simulink model "Usrednjeni_model"  (R2023b)
settings: Solver=ode23t  StartTime=0.0  StopTime=0.001  MaxStep=2.0  RelTol=1e-3
model workspace (MAT data in the model file):
  Upv = 0.5
values from neighbouring files (symbols this model uses):
  pv_data =     [CNC110X69-5.mat]
undefined symbols (not defined in the file or in its folder): Ci, Cu, Ipv0, L, R, RL, T, Uoc_max
libraries: simulink x3, spsBistableLib x1
settings Model: Creator=teo  LastModifiedBy=teo

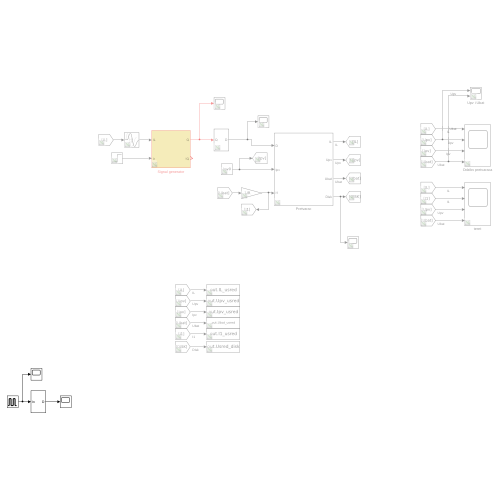
[thumbnail: Simulink's stored preview of the top-level diagram]
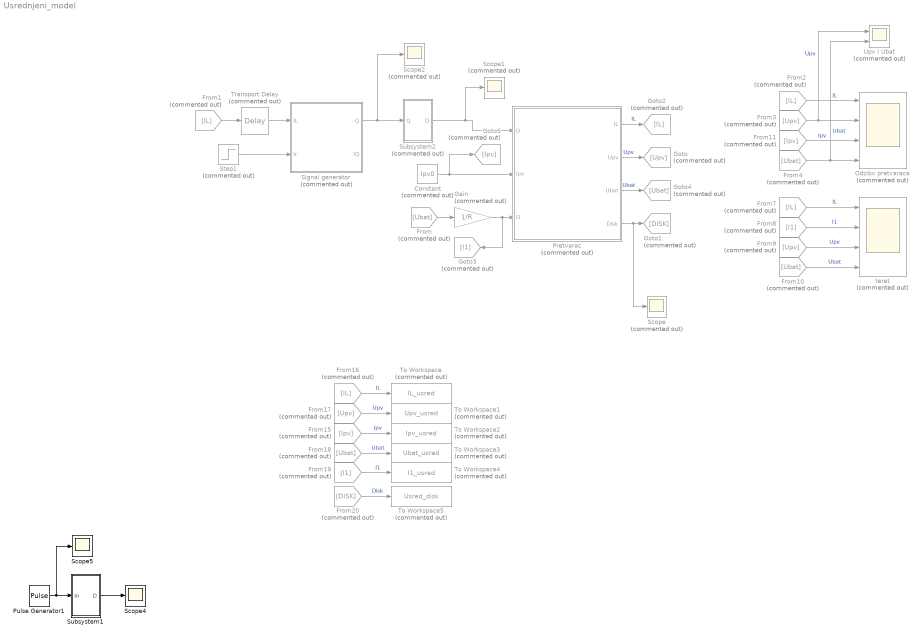
== system Usrednjeni_model ==
  Constant : Constant  Commented=on  Value=Ipv0
  From{,4,10,18} (4 alike) : From  Commented=on  GotoTag=Ubat
  From{1..2,7,16} (4 alike) : From  Commented=on  GotoTag=IL
  From11 : From  Commented=on  GotoTag=Ipv
  From15 : From  Commented=on  GotoTag=Ipv
  From17 : From  Commented=on  GotoTag=Upv
  From19 : From  Commented=on  GotoTag=I1
  From20 : From  Commented=on  GotoTag=DISK
  From3 : From  Commented=on  GotoTag=Upv
  From8 : From  Commented=on  GotoTag=I1
  From9 : From  Commented=on  GotoTag=Upv
  Gain : Gain  Commented=on  Gain=1/R
  Goto : Goto  Commented=on  GotoTag=Upv
  Goto1 : Goto  Commented=on  GotoTag=DISK
  Goto2 : Goto  Commented=on  GotoTag=IL
  Goto3 : Goto  Commented=on  GotoTag=I1
  Goto4 : Goto  Commented=on  GotoTag=Ubat
  Goto5 : Goto  Commented=on  GotoTag=Ipv
  Odzibv pretvaraca : Scope  Commented=on  NumInputPorts=4
  Pretvarac : Subsystem  Commented=on
  Pulse Generator1 : DiscretePulseGenerator  PulseType=Time based  Period=T  PulseWidth=50
  Scope : Scope  Commented=on
  Scope1 : Scope  Commented=on
  Scope2 : Scope  Commented=on
  Scope4 : Scope
  Scope5 : Scope
  Signal generator : Subsystem  Commented=on
  Step1 : Step  Commented=on  Time=0.002  Before=0.1  After=Ipv0 - 0.05  SampleTime=0
  Subsystem1 : Subsystem
  Subsystem2 : Subsystem  Commented=on
  To Workspace : ToWorkspace  Commented=on  VariableName=IL_usred  SaveFormat=Timeseries  SampleTime=-1
  To Workspace1 : ToWorkspace  Commented=on  VariableName=Upv_usred  SaveFormat=Timeseries  SampleTime=-1
  To Workspace2 : ToWorkspace  Commented=on  VariableName=Ipv_usred  SaveFormat=Timeseries  SampleTime=-1
  To Workspace3 : ToWorkspace  Commented=on  VariableName=Ubat_usred  SaveFormat=Timeseries  SampleTime=-1
  To Workspace4 : ToWorkspace  Commented=on  VariableName=I1_usred  SaveFormat=Timeseries  SampleTime=-1
  To Workspace5 : ToWorkspace  Commented=on  VariableName=Usred_disk  SaveFormat=Timeseries  SampleTime=-1
  Transport Delay : TransportDelay  Commented=on  DelayTime=0.0001
  Upv i Ubat : Scope  Commented=on  NumInputPorts=2
  teret : Scope  Commented=on  NumInputPorts=4
  wires:
  Pretvarac/1(IL) -> Goto2/1  "IL"
  Pretvarac/2(Upv) -> Goto/1  "Upv"
  Pretvarac/3(Ubat) -> Goto4/1  "Ubat"
  Pretvarac/4(Disk) -> Scope/1, Goto1/1
  Gain/1 -> Goto3/1, Pretvarac/3(I1)
  From/1 -> Gain/1
  From4/1 -> Upv i Ubat/2, Odzibv pretvaraca/4  "Ubat"
  From2/1 -> Odzibv pretvaraca/1  "IL"
  From3/1 -> Upv i Ubat/1, Odzibv pretvaraca/2  "Upv"
  From8/1 -> teret/2  "I1"
  From10/1 -> teret/4  "Ubat"
  From11/1 -> Odzibv pretvaraca/3  "Ipv"
  From7/1 -> teret/1  "IL"
  From9/1 -> teret/3  "Upv"
  From18/1 -> To Workspace3/1  "Ubat"
  From15/1 -> To Workspace2/1  "Ipv"
  From17/1 -> To Workspace1/1  "Upv"
  From19/1 -> To Workspace4/1  "I1"
  From16/1 -> To Workspace/1  "IL"
  From20/1 -> To Workspace5/1  "Disk"
  Step1/1 -> Signal generator/2(Ir)
  Constant/1 -> Goto5/1, Pretvarac/2(Ipv)
  Subsystem1/1(D) -> Scope4/1
  Pulse Generator1/1 -> Scope5/1, Subsystem1/1(In)
  Signal generator/1(Q) -> Scope2/1, Subsystem2/1(Q)
  Subsystem2/1(D) -> Scope1/1, Pretvarac/1(D)
  Transport Delay/1 -> Signal generator/1(IL)
  From1/1 -> Transport Delay/1

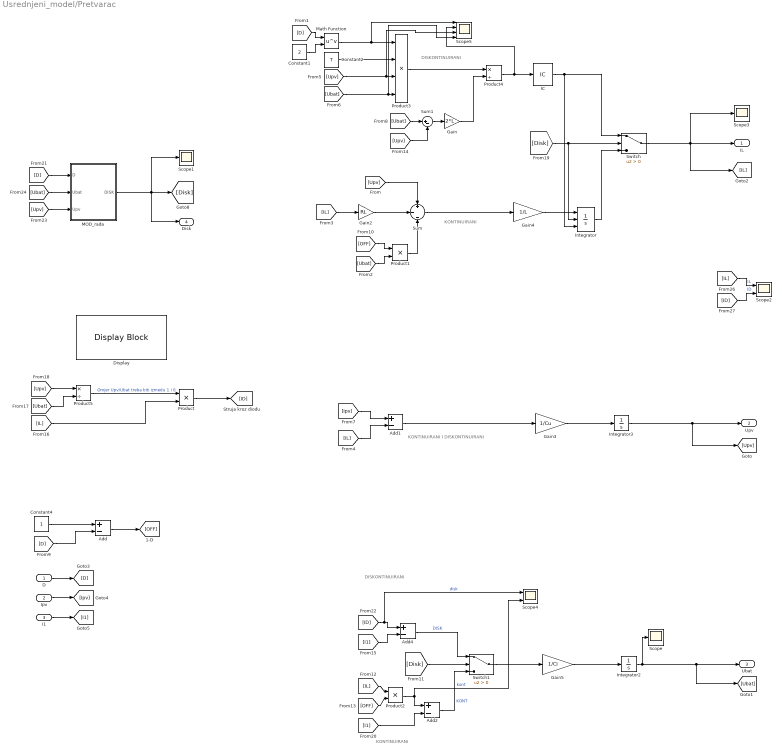
== system Usrednjeni_model/Pretvarac ==
  note: DISKONTINUIRANI
  note: KONTINUIRANI
  note: KONTINUIRANI I DISKONTINUIRANI
  note: KONTINUIRANI
  note: DISKONTINUIRANI
  D : Inport
  Ipv : Inport  Port=2
  I1 : Inport  Port=3
  Add{,1..2,4} (4 alike) : Sum  Inputs=+-
  Constant1 : Constant  Value=2
  Constant2 : Constant  Value=T
  Constant4 : Constant
  Display : DisplayBlock  LabelPosition=Bottom  Transparency=1
  Gain : Gain  Gain=2*L
  Gain2 : Gain  Gain=RL
  Gain3 : Gain  Gain=1/Cu
  Gain4 : Gain  Gain=1/L
  Gain5 : Gain  Gain=1/Ci
  IC : InitialCondition  Value=0.1
  Integrator : Integrator  ExternalReset=falling  InitialConditionSource=external  LimitOutput=on  UpperSaturationLimit=150  LowerSaturationLimit=0
  Integrator2 : Integrator  InitialCondition=0.2  UpperSaturationLimit=Uoc_max + 10  LowerSaturationLimit=0
  Integrator3 : Integrator  InitialCondition=0.1  LimitOutput=on  UpperSaturationLimit=pv_data.Voc  LowerSaturationLimit=0
  MOD_rada : Subsystem
  Math Function : Math  Operator=pow
  Product : Product
  Product1 : Product
  Product2 : Product
  Product3 : Product  Inputs=4
  Product4 : Product  Inputs=*/
  Product5 : Product  Inputs=*/
  Scope : Scope
  Scope1 : Scope
  Scope2 : Scope  NumInputPorts=2
  Scope3 : Scope
  Scope4 : Scope  NumInputPorts=2
  Scope5 : Scope  NumInputPorts=4
  Sum : Sum  Inputs=+|-|-
  Sum1 : Sum  Inputs=|+-
  Switch : Switch  Criteria=u2 > Threshold  SaturateOnIntegerOverflow=off  InputSameDT=off
  Switch1 : Switch  Criteria=u2 > Threshold  SaturateOnIntegerOverflow=off  InputSameDT=off
  IL : Outport
  Upv : Outport  Port=2
  Ubat : Outport  Port=3
  Disk : Outport  Port=4
  wires:
  I1/1 -> [I1]
  [Ipv] -> Add1/1
  D/1 -> [D]
  Ipv/1 -> [Ipv]
  [Upv] -> Sum/1
  [D] -> Add/2
  Constant4/1 -> Add/1
  Product1/1 -> Sum/3
  [OFF] -> Product1/1
  [Ubat] -> Product1/2
  [IL] -> Add1/2
  Sum/1 -> Gain4/1
  Add1/1 -> Gain3/1
  [D] -> Math Function/1
  Constant1/1 -> Math Function/2
  Math Function/1 -> Scope5/1, Product3/1
  Constant2/1 -> Product3/2
  [Upv] -> Scope5/3, Product3/3
  [Ubat] -> Scope5/4, Product3/4
  Product3/1 -> Product4/1
  [Ubat] -> Sum1/1
  [Upv] -> Sum1/2
  Sum1/1 -> Gain/1
  Gain3/1 -> Integrator3/1
  Gain/1 -> Product4/2
  Switch/1 -> Scope3/1, IL/1, [IL]
  Add/1 -> [OFF]
  Gain2/1 -> Sum/2
  [IL] -> Gain2/1
  Gain5/1 -> Integrator2/1
  [D] -> MOD_rada/1(D)
  [Upv] -> MOD_rada/3(Upv)
  [Ubat] -> MOD_rada/2(Ubat)
  Integrator3/1 -> [Upv], Upv/1
  Gain4/1 -> Integrator/1
  Integrator/1 -> Switch/3
  [Disk] -> Integrator/2, Switch/2
  [Upv] -> Product5/1
  [Ubat] -> Product5/2
  [IL] -> Product/2
  Product/1 -> [ID]
  Product5/1 -> Product/1  "Omjer Upv/Ubat treba biti izmedu 1 i 0"
  [ID] -> Scope4/1, Add4/1  "disk"
  [I1] -> Add4/2
  [IL] -> Scope2/1  "IL"
  [ID] -> Scope2/2  "ID"
  IC/1 -> Integrator/3, Switch/1
  Switch1/1 -> Gain5/1
  Add4/1 -> Switch1/1  "DISK"
  [Disk] -> Switch1/2
  [IL] -> Product2/1
  [OFF] -> Product2/2
  Product2/1 -> Add2/1, Scope4/2  "kont"
  [I1] -> Add2/2
  Add2/1 -> Switch1/3  "KONT"
  MOD_rada/1(DISK) -> Disk/1, Scope1/1, [Disk]
  Integrator2/1 -> [Ubat], Ubat/1, Scope/1
  Product4/1 -> Scope5/2, IC/1

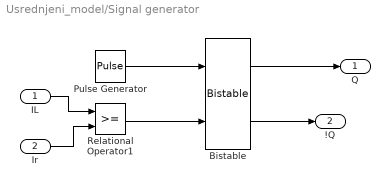
== system Usrednjeni_model/Signal generator ==
  IL : Inport
  Ir : Inport  Port=2
  Bistable : spsBistableLib/Bistable  Qpriority=Set  ic=0  Ts=0
      settings: LibrarySourceBlock=sps_lib/Control/Bistable
  Pulse Generator : DiscretePulseGenerator  PulseType=Time based  Period=T
  Relational Operator1 : RelationalOperator  OutDataTypeStr=boolean  RndMeth=Simplest  InputSameDT=off
  Q : Outport
  !Q : Outport  Port=2
  wires:
  Pulse Generator/1 -> Bistable/1
  Ir/1 -> Relational Operator1/2
  Relational Operator1/1 -> Bistable/2
  IL/1 -> Relational Operator1/1
  Bistable/2 -> !Q/1
  Bistable/1 -> Q/1

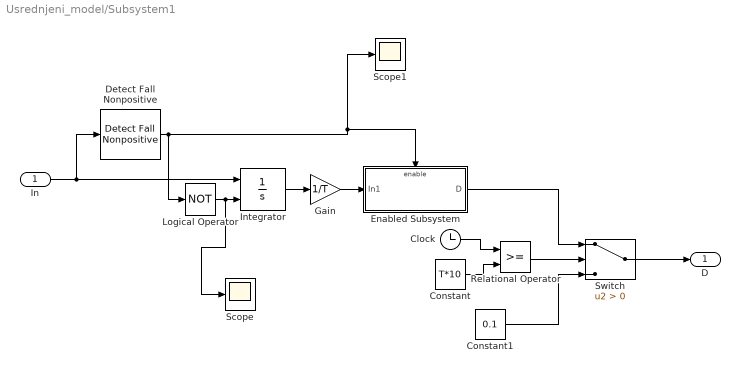
== system Usrednjeni_model/Subsystem1 ==
  In : Inport
  Clock : Clock
  Constant : Constant  Value=T*10
  Constant1 : Constant  Value=0.1
  Detect Fall Nonpositive : simulink/Logic and Bit Operations/Detect Fall Nonpositive  vinit=0  OutDataTypeStr=boolean
  Enabled Subsystem : Subsystem  TreatAsAtomicUnit=on
  Gain : Gain  Gain=1/T
  Integrator : Integrator  ExternalReset=rising
  Logical Operator : Logic  Operator=NOT  AllPortsSameDT=off  OutDataTypeStr=boolean
  Relational Operator : RelationalOperator  OutDataTypeStr=boolean  RndMeth=Simplest  InputSameDT=off
  Scope : Scope
  Scope1 : Scope
  Switch : Switch  Criteria=u2 > Threshold  SaturateOnIntegerOverflow=off  InputSameDT=off
  D : Outport
  wires:
  In/1 -> Integrator/1, Detect Fall Nonpositive/1
  Integrator/1 -> Gain/1
  Gain/1 -> Enabled Subsystem/1(In1)
  Enabled Subsystem/1(D) -> Switch/1
  Switch/1 -> D/1
  Clock/1 -> Relational Operator/1
  Constant/1 -> Relational Operator/2
  Relational Operator/1 -> Switch/2
  Constant1/1 -> Switch/3
  Detect Fall Nonpositive/1 -> Logical Operator/1, Scope1/1, Enabled Subsystem/Enable
  Logical Operator/1 -> Scope/1, Integrator/2

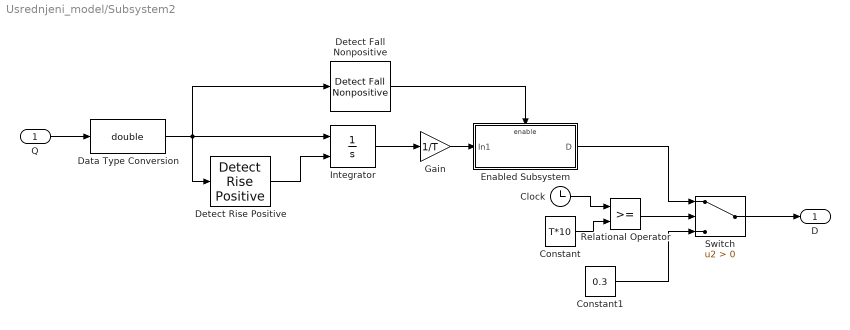
== system Usrednjeni_model/Subsystem2 ==
  Q : Inport
  Clock : Clock
  Constant : Constant  Value=T*10
  Constant1 : Constant  Value=0.3
  Data Type Conversion : DataTypeConversion  OutDataTypeStr=double  SaturateOnIntegerOverflow=off  RndMeth=Floor
  Detect Fall Nonpositive : simulink/Logic and Bit Operations/Detect Fall Nonpositive  vinit=0  OutDataTypeStr=boolean
  Detect Rise Positive : simulink/Logic and Bit Operations/Detect Rise Positive  vinit=0  OutDataTypeStr=boolean
  Enabled Subsystem : Subsystem  TreatAsAtomicUnit=on
  Gain : Gain  Gain=1/T
  Integrator : Integrator  ExternalReset=rising
  Relational Operator : RelationalOperator  OutDataTypeStr=boolean  RndMeth=Simplest  InputSameDT=off
  Switch : Switch  Criteria=u2 > Threshold  SaturateOnIntegerOverflow=off  InputSameDT=off
  D : Outport
  wires:
  Integrator/1 -> Gain/1
  Detect Rise Positive/1 -> Integrator/2
  Gain/1 -> Enabled Subsystem/1(In1)
  Detect Fall Nonpositive/1 -> Enabled Subsystem/Enable
  Enabled Subsystem/1(D) -> Switch/1
  Switch/1 -> D/1
  Clock/1 -> Relational Operator/1
  Constant/1 -> Relational Operator/2
  Relational Operator/1 -> Switch/2
  Constant1/1 -> Switch/3
  Q/1 -> Data Type Conversion/1
  Data Type Conversion/1 -> Detect Rise Positive/1, Detect Fall Nonpositive/1, Integrator/1

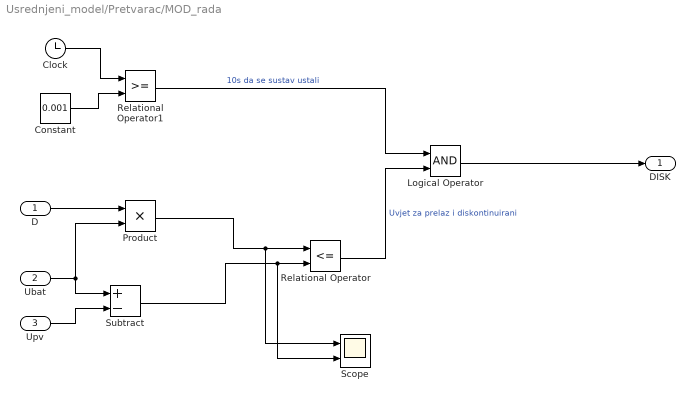
== system Usrednjeni_model/Pretvarac/MOD_rada ==
  D : Inport
  Ubat : Inport  Port=2
  Upv : Inport  Port=3
  Clock : Clock
  Constant : Constant  Value=0.001
  Logical Operator : Logic  AllPortsSameDT=off  OutDataTypeStr=boolean
  Product : Product
  Relational Operator : RelationalOperator  Operator=<=  OutDataTypeStr=boolean  RndMeth=Simplest  InputSameDT=off
  Relational Operator1 : RelationalOperator  OutDataTypeStr=boolean  RndMeth=Simplest  InputSameDT=off
  Scope : Scope  NumInputPorts=2
  Subtract : Sum  Inputs=+-
  DISK : Outport
  wires:
  Ubat/1 -> Product/2, Subtract/1
  Upv/1 -> Subtract/2
  Relational Operator1/1 -> Logical Operator/1  "10s da se sustav ustali"
  Relational Operator/1 -> Logical Operator/2  "Uvjet za prelaz i diskontinuirani"
  Subtract/1 -> Scope/2, Relational Operator/2
  Product/1 -> Scope/1, Relational Operator/1
  Logical Operator/1 -> DISK/1
  Clock/1 -> Relational Operator1/1
  Constant/1 -> Relational Operator1/2
  D/1 -> Product/1

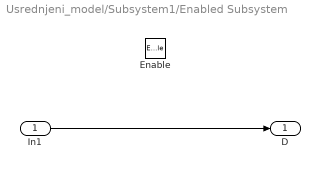
== system Usrednjeni_model/Subsystem1/Enabled Subsystem ==
  In1 : Inport
  Enable : EnablePort
  D : Outport
  wires:
  In1/1 -> D/1

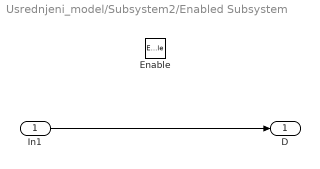
== system Usrednjeni_model/Subsystem2/Enabled Subsystem ==
  In1 : Inport
  Enable : EnablePort
  D : Outport
  wires:
  In1/1 -> D/1
